simulink model "Model_pf_regulacije"  (R2024a)
settings: Solver=VariableStepAuto  StartTime=0.0  StopTime=Tsim  RelTol=1e-3
values from neighbouring files (symbols this model uses):
  Cv = [c1 c0]    [Model_pf_regulacije_eng.m]
  Fn = 50    [Model_pf_regulacije_eng.m]
  Lv = [l1 l0]    [Model_pf_regulacije_eng.m]
  n_LG2_CHM = 13    [Model_pf_regulacije_eng.m]
  n_LG2_LG3 = 2    [Model_pf_regulacije_eng.m]
  n_LG3_CHM = 6    [Model_pf_regulacije_eng.m]
  n_LG3_LG4 = 2    [Model_pf_regulacije_eng.m]
  n_LG4_CHM = 8    [Model_pf_regulacije_eng.m]
  P_LG31loc = 5e6    (= 5000000)    [Model_pf_regulacije_eng.m]
  PSStype = 1    [Model_pf_regulacije_eng.m]
  Rv = [r1 r0]    [Model_pf_regulacije_eng.m]
  t_ispad_LG31 = 100    [Model_pf_regulacije_eng.m]
  t_ispad_voda_LG2_LG3 = 1e6    (= 1000000)    [Model_pf_regulacije_eng.m]
  t_povecanje_potrosnje = 1e6    (= 1000000)    [Model_pf_regulacije_eng.m]
  Ts = 50e-6    (= 5e-05)    [Model_pf_regulacije_eng.m]
  Vg = 13.8e3    (= 13800)    [Model_pf_regulacije_eng.m]
  Vrms = 230e3    (= 230000)    [Model_pf_regulacije_eng.m]
undefined symbols (not defined in the file or in its folder): D1, Delta
libraries: spsThreePhaseParallelRLCLoadLib x6, spsDistributedParametersLineLib x5, spsThreePhaseTransformerTwoWindingsLib x4, spsSynchronousMachinepuStandardLib x4, spsRMSLib x4, spsExcitationSystemLib x4, spsHydraulicTurbineandGovernorLib x4, spsGenericPowerSystemStabilizerLib x4, spsMultiBandPowerSystemStabilizerLib x4, spsThreePhaseBreakerLib x3, spsThreePhaseSeriesRLCLoadLib x2, dspstat3 x2
(part 1 of 2)
settings Model: Creator=nesat  LastModifiedBy=nesat

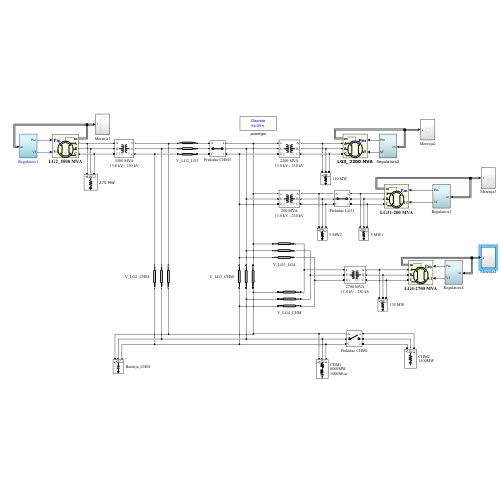
[thumbnail: Simulink's stored preview of the top-level diagram]
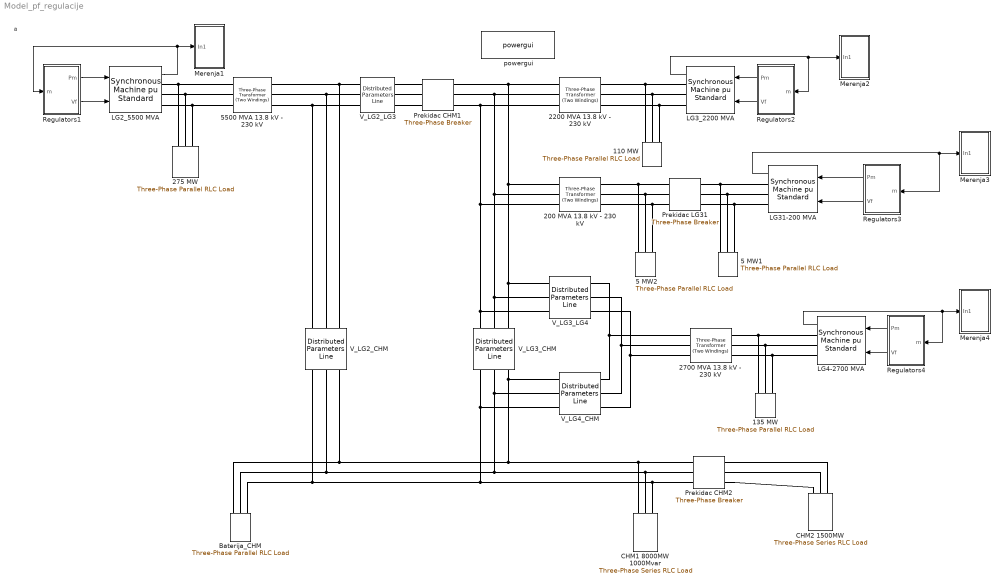
== system Model_pf_regulacije ==
  note: a
  110 MW : spsThreePhaseParallelRLCLoadLib/Three-Phase Parallel RLC Load  LConnTagsString=A|B|C  Configuration=Y (grounded)  NominalVoltage=(13800)*1  Vabc=[1e3 1e3 1e3]  Vabcp=[1e3 1e3 1e3]  NominalFrequency=Fn  UnbalancedPower=off  ActivePower=110000000  InductivePower=0  CapacitivePower=0  Pabc=[10e3 9e3 11e3]  QLabc=[100 90 110]  QCabc=[100 90 110]  Pabcp=[10e3 9e3 11e3]  QLabcp=[100 90 110]  QCabcp=[100 90 110]  Measurements=None  LoadType=constant PQ
  135 MW : spsThreePhaseParallelRLCLoadLib/Three-Phase Parallel RLC Load  LConnTagsString=A|B|C  Configuration=Y (grounded)  NominalVoltage=(13800)*1  Vabc=[1e3 1e3 1e3]  Vabcp=[1e3 1e3 1e3]  NominalFrequency=Fn  UnbalancedPower=off  ActivePower=135000000  InductivePower=0  CapacitivePower=0  Pabc=[10e3 9e3 11e3]  QLabc=[100 90 110]  QCabc=[100 90 110]  Pabcp=[10e3 9e3 11e3]  QLabcp=[100 90 110]  QCabcp=[100 90 110]  Measurements=None  LoadType=constant PQ
  200 MVA 13.8 kV - 230 kV : spsThreePhaseTransformerTwoWindingsLib/Three-Phase Transformer (Two Windings)  Winding1Connection=Delta (D1)  Winding2Connection=Yg  CoreType=Three single-phase transformers  SetSaturation=off  Hysteresis=off  DataFile='basic_model'  SetInitialFlux=off  Measurements=None  UNITS=pu  NominalPower=[ 200e6 Fn ]  Winding1="[ Vg 0.002  0.0]"  Winding2=[ Vrms 0.002 0.12]  Rm=500  Lm=500  L0=0.5  Saturation="[ 0,0  ;  0.005,1.2  ;  1.0,1.4 ]"  InitialFluxes=[ 0.8 , -0.8 , 0.7 ]  BreakLoop=off  DiscreteSolver=Trapezoidal iterative  DataType=off  TransfoNumber=0
  2200 MVA 13.8 kV - 230 kV : spsThreePhaseTransformerTwoWindingsLib/Three-Phase Transformer (Two Windings)  Winding1Connection=Delta (D1)  Winding2Connection=Yg  CoreType=Three single-phase transformers  SetSaturation=off  Hysteresis=off  DataFile='basic_model'  SetInitialFlux=off  Measurements=None  UNITS=pu  NominalPower=[ 2200e6 Fn ]  Winding1="[ Vg 0.002  0.0]"  Winding2=[ Vrms 0.002 0.12]  Rm=500  Lm=500  L0=0.5  Saturation="[ 0,0  ;  0.005,1.2  ;  1.0,1.4 ]"  InitialFluxes=[ 0.8 , -0.8 , 0.7 ]  BreakLoop=off  DiscreteSolver=Trapezoidal iterative  DataType=off  TransfoNumber=0
  2700 MVA 13.8 kV - 230 kV : spsThreePhaseTransformerTwoWindingsLib/Three-Phase Transformer (Two Windings)  Winding1Connection=Delta (D1)  Winding2Connection=Yg  CoreType=Three single-phase transformers  SetSaturation=off  Hysteresis=off  DataFile='basic_model'  SetInitialFlux=off  Measurements=None  UNITS=pu  NominalPower=[ 2700e6 Fn ]  Winding1="[ Vg 0.002  0.0]"  Winding2=[ Vrms 0.002 0.12]  Rm=500  Lm=500  L0=0.5  Saturation="[ 0,0  ;  0.005,1.2  ;  1.0,1.4 ]"  InitialFluxes=[ 0.8 , -0.8 , 0.7 ]  BreakLoop=off  DiscreteSolver=Trapezoidal iterative  DataType=off  TransfoNumber=0
  275 MW : spsThreePhaseParallelRLCLoadLib/Three-Phase Parallel RLC Load  LConnTagsString=A|B|C  Configuration=Y (grounded)  NominalVoltage=(13800)*1  Vabc=[1e3 1e3 1e3]  Vabcp=[1e3 1e3 1e3]  NominalFrequency=Fn  UnbalancedPower=off  ActivePower=275000000  InductivePower=0  CapacitivePower=0  Pabc=[10e3 9e3 11e3]  QLabc=[100 90 110]  QCabc=[100 90 110]  Pabcp=[10e3 9e3 11e3]  QLabcp=[100 90 110]  QCabcp=[100 90 110]  Measurements=None  LoadType=constant PQ
  5 MW1 : spsThreePhaseParallelRLCLoadLib/Three-Phase Parallel RLC Load  LConnTagsString=A|B|C  Configuration=Y (grounded)  NominalVoltage=(13800)*1  Vabc=[1e3 1e3 1e3]  Vabcp=[1e3 1e3 1e3]  NominalFrequency=Fn  UnbalancedPower=off  ActivePower=110000000  InductivePower=0  CapacitivePower=0  Pabc=[10e3 9e3 11e3]  QLabc=[100 90 110]  QCabc=[100 90 110]  Pabcp=[10e3 9e3 11e3]  QLabcp=[100 90 110]  QCabcp=[100 90 110]  Measurements=None  LoadType=constant PQ
  5 MW2 : spsThreePhaseParallelRLCLoadLib/Three-Phase Parallel RLC Load  LConnTagsString=A|B|C  Configuration=Y (grounded)  NominalVoltage=(13749.3)*1  Vabc=[1e3 1e3 1e3]  Vabcp=[1e3 1e3 1e3]  NominalFrequency=Fn  UnbalancedPower=off  ActivePower=110000000  InductivePower=0  CapacitivePower=0  Pabc=[10e3 9e3 11e3]  QLabc=[100 90 110]  QCabc=[100 90 110]  Pabcp=[10e3 9e3 11e3]  QLabcp=[100 90 110]  QCabcp=[100 90 110]  Measurements=None  LoadType=constant PQ
  5500 MVA 13.8 kV - 230 kV : spsThreePhaseTransformerTwoWindingsLib/Three-Phase Transformer (Two Windings)  Winding1Connection=Delta (D1)  Winding2Connection=Yg  CoreType=Three single-phase transformers  SetSaturation=off  Hysteresis=off  DataFile='basic_model'  SetInitialFlux=off  Measurements=None  UNITS=pu  NominalPower=[ 5500e6 Fn ]  Winding1="[ Vg 0.002  0.0]"  Winding2=[ Vrms 0.002 0.12]  Rm=500  Lm=500  L0=0.5  Saturation="[ 0,0  ;  0.005,1.2  ;  1.0,1.4 ]"  InitialFluxes=[ 0.8 , -0.8 , 0.7 ]  BreakLoop=off  DiscreteSolver=Trapezoidal iterative  DataType=off  TransfoNumber=0
  Baterija_CHM : spsThreePhaseParallelRLCLoadLib/Three-Phase Parallel RLC Load  LConnTagsString=A|B|C  Configuration=Y (grounded)  NominalVoltage=Vrms  Vabc=[1e3 1e3 1e3]  Vabcp=[1e3 1e3 1e3]  NominalFrequency=Fn  UnbalancedPower=off  ActivePower=0  InductivePower=0  CapacitivePower=2200000000  Pabc=[10e3 9e3 11e3]  QLabc=[100 90 110]  QCabc=[100 90 110]  Pabcp=[10e3 9e3 11e3]  QLabcp=[100 90 110]  QCabcp=[100 90 110]  Measurements=None  LoadType=constant Z
  CHM1 8000MW 1000Mvar : spsThreePhaseSeriesRLCLoadLib/Three-Phase Series RLC Load  LConnTagsString=A|B|C  Configuration=Y (grounded)  NominalVoltage=Vrms  Vabc=[1e3 1e3 1e3]  Vabcp=[1e3 1e3 1e3]  NominalFrequency=Fn  UnbalancedPower=off  ActivePower=8000000000  InductivePower=1000000000  CapacitivePower=0  Pabc=[10e3 9e3 11e3]  QLabc=[100 90 110]  QCabc=[100 90 110]  Pabcp=[10e3 9e3 11e3]  QLabcp=[100 90 110]  QCabcp=[100 90 110]  Measurements=None  LoadType=constant Z
  CHM2 1500MW : spsThreePhaseSeriesRLCLoadLib/Three-Phase Series RLC Load  LConnTagsString=A|B|C  Configuration=Y (grounded)  NominalVoltage=Vrms  Vabc=[1e3 1e3 1e3]  Vabcp=[1e3 1e3 1e3]  NominalFrequency=Fn  UnbalancedPower=off  ActivePower=1500000000  InductivePower=0  CapacitivePower=0  Pabc=[10e3 9e3 11e3]  QLabc=[100 90 110]  QCabc=[100 90 110]  Pabcp=[10e3 9e3 11e3]  QLabcp=[100 90 110]  QCabcp=[100 90 110]  Measurements=None  LoadType=constant Z
  LG2_5500 MVA : spsSynchronousMachinepuStandardLib/Synchronous Machine pu Standard  PresetModel=No  MechanicalLoad=Mechanical power Pm  ShowDetailedParameters=on  RotorType=Salient-pole  Units=per unit standard parameters  MeasurementBus=off  NominalParameters="[5500E6  Vg   Fn ]"  Reactances1=[ 31 32 33 34 35 36 37 ]  Reactances2=[ 1.305, 0.296, 0.252, 0.474, 0.243, 0.18 ]  dAxisTimeConstants=Short-circuit  qAxisTimeConstants=Open-circuit  TimeConstants1=[]  TimeConstants2=[]  TimeConstants3=[]  TimeConstants4=[]  TimeConstants5=[ 1.01, 0.053, 0.1 ]  TimeConstants6=[]  TimeConstants7=[]  TimeConstants8=[]  StatorResistance=2.8544e-3  Mechanical="[ 4.1  0  32]"  PolePairs=32  InitialConditions=[0 -70.1006 0.783509 0.783509 0.783509 -3.33907 -123.339 116.661 1.34578]  SetSaturation=off  Saturation=[0.6404,0.7127,0.8441,0.9214,0.9956,1.082,1.19,1.316,1.457;0.7,0.7698,0.8872,0.9466,0.9969,1.046,1.1,1.151,1.201]  LoadFlowParameters=[2 4000000000 0 0 0]  TsPowergui=0  TsBlock=-1  IterativeModel=Trapezoidal non iterative  IterativeDiscreteModel=Trapezoidal non iterative  BusType=swing  Pref=0  Qref=0  Qmin=-Inf  Qmax=Inf  PLF=0  QLF=0
  LG31-200 MVA : spsSynchronousMachinepuStandardLib/Synchronous Machine pu Standard  PresetModel=No  MechanicalLoad=Mechanical power Pm  ShowDetailedParameters=on  RotorType=Salient-pole  Units=per unit standard parameters  MeasurementBus=off  NominalParameters="[200E6  Vg   Fn ]"  Reactances1=[ 31 32 33 34 35 36 37 ]  Reactances2=[ 1.305, 0.296, 0.252, 0.474, 0.243, 0.18 ]  dAxisTimeConstants=Short-circuit  qAxisTimeConstants=Open-circuit  TimeConstants1=[]  TimeConstants2=[]  TimeConstants3=[]  TimeConstants4=[]  TimeConstants5=[ 1.01, 0.053, 0.1 ]  TimeConstants6=[]  TimeConstants7=[]  TimeConstants8=[]  StatorResistance=2.8544e-3  Mechanical="[ 3.2  0  32]"  PolePairs=32  InitialConditions=[0 -75.957 0.900232 0.900232 0.900232 -10.1077 -130.108 109.892 1.40453]  SetSaturation=off  Saturation=[0.6404,0.7127,0.8441,0.9214,0.9956,1.082,1.19,1.316,1.457;0.7,0.7698,0.8872,0.9466,0.9969,1.046,1.1,1.151,1.201]  LoadFlowParameters=[1 180000000 0 0 0]  TsPowergui=0  TsBlock=-1  IterativeModel=Trapezoidal non iterative  IterativeDiscreteModel=Trapezoidal non iterative  BusType=PV  Pref=180000000  Qref=0  Qmin=-Inf  Qmax=Inf  PLF=0  QLF=0
  LG3_2200 MVA : spsSynchronousMachinepuStandardLib/Synchronous Machine pu Standard  PresetModel=No  MechanicalLoad=Mechanical power Pm  ShowDetailedParameters=on  RotorType=Salient-pole  Units=per unit standard parameters  MeasurementBus=off  NominalParameters="[2200E6  Vg   Fn ]"  Reactances1=[ 31 32 33 34 35 36 37 ]  Reactances2=[ 1.305, 0.296, 0.252, 0.474, 0.243, 0.18 ]  dAxisTimeConstants=Short-circuit  qAxisTimeConstants=Open-circuit  TimeConstants1=[]  TimeConstants2=[]  TimeConstants3=[]  TimeConstants4=[]  TimeConstants5=[ 1.01, 0.053, 0.1 ]  TimeConstants6=[]  TimeConstants7=[]  TimeConstants8=[]  StatorResistance=2.8544e-3  Mechanical="[ 3.2  0  32]"  PolePairs=32  InitialConditions=[0 -71.4065 0.819807 0.819807 0.819807 -5.69934 -125.699 114.301 1.37781]  SetSaturation=off  Saturation=[0.6404,0.7127,0.8441,0.9214,0.9956,1.082,1.19,1.316,1.457;0.7,0.7698,0.8872,0.9466,0.9969,1.046,1.1,1.151,1.201]  LoadFlowParameters=[1 1800000000 0 0 0]  TsPowergui=0  TsBlock=-1  IterativeModel=Trapezoidal non iterative  IterativeDiscreteModel=Trapezoidal non iterative  BusType=PV  Pref=1800000000  Qref=0  Qmin=-Inf  Qmax=Inf  PLF=0  QLF=0
  LG4-2700 MVA : spsSynchronousMachinepuStandardLib/Synchronous Machine pu Standard  PresetModel=No  MechanicalLoad=Mechanical power Pm  ShowDetailedParameters=on  RotorType=Salient-pole  Units=per unit standard parameters  MeasurementBus=off  NominalParameters="[2700E6  Vg   Fn ]"  Reactances1=[ 31 32 33 34 35 36 37 ]  Reactances2=[ 1.305, 0.296, 0.252, 0.474, 0.243, 0.18 ]  dAxisTimeConstants=Short-circuit  qAxisTimeConstants=Open-circuit  TimeConstants1=[]  TimeConstants2=[]  TimeConstants3=[]  TimeConstants4=[]  TimeConstants5=[ 1.01, 0.053, 0.1 ]  TimeConstants6=[]  TimeConstants7=[]  TimeConstants8=[]  StatorResistance=2.8544e-3  Mechanical="[ 3.7  0  32]"  PolePairs=32  InitialConditions=[0 -69.3817 0.928059 0.928059 0.928059 -6.28858 -126.289 113.711 1.4708]  SetSaturation=off  Saturation=[0.6404,0.7127,0.8441,0.9214,0.9956,1.082,1.19,1.316,1.457;0.7,0.7698,0.8872,0.9466,0.9969,1.046,1.1,1.151,1.201]  LoadFlowParameters=[1 2500000000 0 0 0]  TsPowergui=0  TsBlock=-1  IterativeModel=Trapezoidal non iterative  IterativeDiscreteModel=Trapezoidal non iterative  BusType=PV  Pref=2500000000  Qref=0  Qmin=-Inf  Qmax=Inf  PLF=0  QLF=0
  Merenja1 : Subsystem
  Merenja2 : Subsystem
  Merenja3 : Subsystem
  Merenja4 : Subsystem
  Prekidac CHM1 : spsThreePhaseBreakerLib/Three-Phase Breaker  InitialState=closed  SwitchA=on  SwitchB=on  SwitchC=on  SwitchTimes=[t_ispad_voda_LG2_LG3]  External=off  BreakerResistance=0.01  SnubberResistance=inf  SnubberCapacitance=inf  Measurements=None
  Prekidac CHM2 : spsThreePhaseBreakerLib/Three-Phase Breaker  InitialState=open  SwitchA=on  SwitchB=on  SwitchC=on  SwitchTimes=[t_povecanje_potrosnje]  External=off  BreakerResistance=0.01  SnubberResistance=inf  SnubberCapacitance=inf  Measurements=None
  Prekidac LG31 : spsThreePhaseBreakerLib/Three-Phase Breaker  InitialState=closed  SwitchA=on  SwitchB=on  SwitchC=on  SwitchTimes=[t_ispad_LG31]  External=off  BreakerResistance=0.01  SnubberResistance=inf  SnubberCapacitance=inf  Measurements=None
  Regulators1 : Subsystem
  Regulators2 : Subsystem
  Regulators3 : Subsystem
  Regulators4 : Subsystem
  V_LG2_CHM : spsDistributedParametersLineLib/Distributed Parameters Line  Phases=3  Length=d_LG2_CHM  Frequency=Fn  Resistance=Rv/n_LG2_CHM  Inductance=Lv/n_LG2_CHM  Capacitance=Cv*n_LG2_CHM  x1=[-0.0004 -4.92231625974316e-10 0 0;-0.00035 -4.9297484247355e-10 0 0;-0.0003 -4.93596424806945e-10 174298.798867466 -148541.05620319;-0.00025 -4.9409621960836e-10 176610.478606358 -145784.962686328;-0.0002 -4.94474103560907e-10 178878.582352334 -142992.898911351;-0.00015 -4.94729983427376e-10 181102.550484731 -140165.553778216;-0.0001 -4.94863796073237e-10 183281.834272692 -137303.624892029;-5e-05 -4.94875508482223e-10 185415.896010552 -134407.818390917]  x2=[-0.0004 2.36773299637199e-10 0 0;-0.00035 2.32836541357427e-10 0 0;-0.0003 2.28842334145082e-10 144026.029759485 -176441.794650633;-0.00025 2.24791663511028e-10 146779.690253438 -174157.764140718;-0.0002 2.20685528897633e-10 149497.135055132 -171830.76280848;-0.00015 2.16524943432171e-10 152177.693675726 -169461.364806678;-0.0001 2.12310933676849e-10 154820.704727488 -167050.154748815;-5e-05 2.08044539375519e-10 157425.516086991 -164597.727564892]  x3=[-0.0004 3.21876795891022e-11 0 0;-0.00035 3.32508643823564e-11 0 0;-0.0003 3.43058450223675e-11 -6703.30163476618 5237.16864274642;-0.00025 3.53523612084488e-11 -6784.73607008563 5131.23180111232;-0.0002 3.63901547283906e-11 -6864.49647330198 5024.02890481155;-0.00015 3.74189695221708e-11 -6942.5631647292 4915.58640455469;-0.0001 3.84385517451334e-11 -7018.91688257933 4805.931056906;-5e-05 3.94486498306213e-11 -7093.53878771499 4695.08991768171]  x4=[-0.0004 -4.06922002783782e-11 0 0;-0.00035 -4.20487159660441e-11 0 0;-0.0003 -4.33948567622339e-11 17021.6965149512 -16716.63043995;-0.00025 -4.47302905268488e-11 17282.1696226858 -16447.2030111636;-0.0002 -4.60546877615899e-11 17538.3786136646 -16173.7174811389;-0.00015 -4.73677216912569e-11 17790.2602721529 -15896.2413283383;-0.0001 -4.8669068344375e-11 18037.7524501204 -15614.8430158504;-5e-05 -4.995840663313e-11 18280.7940825755 -15329.5919744984]  x5=0.000365161017096251  V1=ones(3,3)  V2=ones(3,3)  I1=ones(3,3)  I2=ones(3,3)  nHarmo=1  Measurements=None  Decoupling=on  VsMag0=[186984.075518439 186983.986127739 186984.058818565]  VrMag0=[185966.39343063 185966.327411481 185966.338035223]  VsAngle0=[24.9616648723654 -95.0383252221643 144.961693546538]  VrAngle0=[14.6240938483193 -105.375914115677 134.624107481573]  IsMag0=[6982.19028183256 6982.21077254924 6982.2073947194]  IrMag0=[19582.2755022873 19582.289528592 19582.2917657676]  IsAngle0=[-152.599793624276 87.400271448419 -32.5999067067536]  IrAngle0=[20.9180760110638 -99.0818927363708 140.918056096077]
      settings: AttributesFormatString=\n
  V_LG2_LG3 : spsDistributedParametersLineLib/Distributed Parameters Line  Phases=3  Length=d_LG2_LG3  Frequency=Fn  Resistance=Rv/n_LG2_LG3  Inductance=Lv/n_LG2_LG3  Capacitance=Cv*n_LG2_LG3  x1=[-0.0002 -4.94474103560907e-10 0 0;-0.00015 -4.94729983427376e-10 181102.550484731 -140165.553778216;-0.0001 -4.94863796073237e-10 183281.834272692 -137303.624892029;-5e-05 -4.94875508482223e-10 185415.896010552 -134407.818390917]  x2=[-0.0002 -7.7953967209642e-10 0 0;-0.00015 -7.86855540206448e-10 175151.457634006 -147384.64347033;-0.0001 -7.93977263485902e-10 177444.868089399 -144615.299555331;-5e-05 -8.00903084756128e-10 179694.496678755 -141810.273979092]  x3=[-0.0002 1.33778643921854e-11 0 0;-0.00015 1.31674782162147e-11 -28.2189110152237 -142.274491350519;-0.0001 1.29538431620234e-11 -25.9806898373746 -142.700175699615;-5e-05 1.27370119408644e-11 -23.7360583130655 -143.090650915626]  x4=[-0.0002 -1.7897483501798e-11 0 0;-0.00015 -1.77244134939981e-11 1861.28121044207 -1403.22806397395;-0.0001 -1.75469702523846e-11 1883.09255919525 -1373.81920400992;-5e-05 -1.73651975584223e-11 1904.43928303676 -1344.0713747142]  x5=0.000182580508548125  V1=ones(3,3)  V2=ones(3,3)  I1=ones(3,3)  I2=ones(3,3)  nHarmo=1  Measurements=None  Decoupling=on  VsMag0=[186984.075518439 186983.986127739 186984.058818565]  VrMag0=[186905.178173425 186905.084989887 186905.161229939]  VsAngle0=[24.9616648723654 -95.0383252221643 144.961693546538]  VrAngle0=[22.6203950553895 -97.3795944499093 142.620425041114]  IsMag0=[118.740998777895 118.740595365614 118.741154186562]  IrMag0=[1908.23825342973 1908.23711991417 1908.23756444361]  IsAngle0=[-38.5186191165268 -158.518420141088 81.4816489491208]  IrAngle0=[25.6871839847176 -94.3128202530022 145.687211340485]
      settings: AttributesFormatString=\n
  V_LG3_CHM : spsDistributedParametersLineLib/Distributed Parameters Line  Phases=3  Length=d_LG3_CHM  Frequency=Fn  Resistance=Rv/n_LG3_CHM  Inductance=Lv/n_LG3_CHM  Capacitance=Cv*n_LG3_CHM  x1=[-0.0003 3.60679163287581e-10 0 0;-0.00025 3.46849489679935e-10 170426.301829629 -152806.935817911;-0.0002 3.32934236150731e-10 172805.464821387 -150111.142456335;-0.00015 3.18936836080559e-10 175141.990650445 -147378.311416519;-0.0001 3.04860743118438e-10 177435.302814015 -144609.116983631;-5e-05 2.90709430329682e-10 179684.835471637 -141804.242414959]  x2=[-0.0003 5.63637905808929e-11 0 0;-0.00025 5.18487152588664e-11 146779.690253438 -174157.764140718;-0.0002 4.73208470421787e-11 149497.135055132 -171830.76280848;-0.00015 4.27813031145603e-11 152177.693675726 -169461.364806678;-0.0001 3.82312035405489e-11 154820.704727488 -167050.154748815;-5e-05 3.36716709891296e-11 157425.516086992 -164597.727564892]  x3=[-0.0003 -5.17988986960856e-11 0 0;-0.00025 -5.21005495720223e-11 -3261.95177657882 2594.96524324426;-0.0002 -5.23893454169493e-11 -3302.30898560715 2543.40867748096;-0.00015 -5.26652149748133e-11 -3341.85139930679 2491.22456368434;-0.0001 -5.29280901789288e-11 -3380.56926117886 2438.42577750362;-5e-05 -5.31779061687727e-11 -3418.45301817026 2385.02534624926]  x4=[-0.0003 5.38997922352836e-11 0 0;-0.00025 5.41154066451993e-11 8069.93383069662 -7880.48555179821;-0.0002 5.43176688882715e-11 8192.71927209322 -7752.75638122329;-0.00015 5.45065290593182e-11 8313.48328259971 -7623.11433401827;-0.0001 5.46819405599183e-11 8432.19606550355 -7491.59139741845;-5e-05 5.48438601099086e-11 8548.82833020188 -7358.2200227404]  x5=0.000273870762822188  V1=ones(3,3)  V2=ones(3,3)  I1=ones(3,3)  I2=ones(3,3)  nHarmo=1  Measurements=None  Decoupling=on  VsMag0=[186895.934962322 186895.841784948 186895.91802478]  VrMag0=[185966.39343063 185966.327411481 185966.338035223]  VsAngle0=[22.6200820806876 -97.3799074230796 142.620112066765]  VrAngle0=[14.6240938483193 -105.375914115677 134.624107481573]  IsMag0=[3416.77743069497 3416.79081502547 3416.789329226]  IrMag0=[9245.99519366939 9246.00534372241 9246.00684286608]  IsAngle0=[-154.003037127926 85.997063683 -34.0031810934756]  IrAngle0=[20.1805111179014 -99.819441840853 140.180480167284]
      settings: AttributesFormatString=\n
  V_LG3_LG4 : spsDistributedParametersLineLib/Distributed Parameters Line  Phases=3  Length=d_LG3_LG4  Frequency=Fn  Resistance=Rv/n_LG3_LG4  Inductance=Lv/n_LG3_LG4  Capacitance=Cv*n_LG3_LG4  x1=[-0.0002 3.32934236150731e-10 0 0;-0.00015 3.18936836080559e-10 175141.990650445 -147378.311416519;-0.0001 3.04860743118438e-10 177435.302814015 -144609.116983631;-5e-05 2.90709430329682e-10 179684.835471637 -141804.242414959]  x2=[-0.0002 1.21043284557454e-10 0 0;-0.00015 1.09009725018709e-10 172295.654093928 -150519.718237425;-0.0001 9.69492689614629e-11 174638.661520085 -147794.848187023;-5e-05 8.48648921227839e-11 176938.579469686 -145033.511969331]  x3=[-0.0002 -6.1608129553596e-12 0 0;-0.00015 -6.39604605721854e-12 478.611469515026 -493.959673085078;-0.0001 -6.62970103041895e-12 486.311664006773 -486.380949799821;-5e-05 -6.86172022409245e-12 493.891868372263 -478.682219293075]  x4=[-0.0002 5.42735736797522e-12 0 0;-0.00015 5.47118398448572e-12 1307.12976761467 -1104.73436688628;-0.0001 5.51366066821513e-12 1324.32048212396 -1084.06665754206;-5e-05 5.55477693867734e-12 1341.18444037052 -1063.13147097132]  x5=0.000182580508548125  V1=ones(3,3)  V2=ones(3,3)  I1=ones(3,3)  I2=ones(3,3)  nHarmo=1  Measurements=None  Decoupling=on  VsMag0=[186895.934962322 186895.841784948 186895.91802478]  VrMag0=[186801.151920291 186801.129926176 186801.036069883]  VsAngle0=[22.6200820806876 -97.3799074230796 142.620112066765]  VrAngle0=[21.5591107129978 -98.4409264229707 141.559097987269]  IsMag0=[563.084208908888 563.067141562085 563.065053621451]  IrMag0=[1401.04156139632 1401.05913786973 1401.05906764344]  IsAngle0=[16.7953210422352 -103.205926979985 136.796201085146]  IrAngle0=[22.4971326327252 -97.502455694665 142.496715985794]
      settings: AttributesFormatString=\n
  V_LG4_CHM : spsDistributedParametersLineLib/Distributed Parameters Line  Phases=3  Length=d_LG4_CHM  Frequency=Fn  Resistance=Rv/n_LG4_CHM  Inductance=Lv/n_LG4_CHM  Capacitance=Cv*n_LG4_CHM  x1=[-0.00025 1.33332411004425e-10 0 0;-0.0002 1.21271715136788e-10 169910.135293239 -153207.449799628;-0.00015 1.09181097288068e-10 172295.654093928 -150519.718237425;-0.0001 9.70635406373038e-11 174638.661520085 -147794.848187023;-5e-05 8.49220350102806e-11 176938.579469686 -145033.511969331]  x2=[-0.00025 5.18487152588664e-11 0 0;-0.0002 4.73208470421787e-11 149497.135055132 -171830.76280848;-0.00015 4.27813031145603e-11 152177.693675726 -169461.364806678;-0.0001 3.82312035405489e-11 154820.704727488 -167050.154748815;-5e-05 3.36716709891296e-11 157425.516086992 -164597.727564892]  x3=[-0.00025 -6.35851188186883e-11 0 0;-0.0002 -6.37198904871654e-11 -4698.16701989244 3704.41558440375;-0.00015 -6.38389402261261e-11 -4755.77476748485 3630.1627630419;-0.0001 -6.39422386618285e-11 -4812.20909881558 3555.01425333756;-5e-05 -6.40297603069293e-11 -4867.4560895578 3478.98859706102]  x4=[-0.00025 6.15787065574911e-11 0 0;-0.0002 6.13911826988325e-11 11198.9922638145 -10684.0251642951;-0.00015 6.1188511484459e-11 11365.4290381183 -10506.8007786139;-0.0001 6.097074292046e-11 11529.0615628715 -10326.9839970573;-5e-05 6.07379307379701e-11 11689.8494641972 -10144.6191867253]  x5=0.000228225635685157  V1=ones(3,3)  V2=ones(3,3)  I1=ones(3,3)  I2=ones(3,3)  nHarmo=1  Measurements=None  Decoupling=on  VsMag0=[186801.151920291 186801.129926176 186801.036069883]  VrMag0=[185966.39343063 185966.327411481 185966.338035223]  VsAngle0=[21.5591107129978 -98.4409264229707 141.559097987269]  VrAngle0=[14.6240938483193 -105.375914115677 134.624107481573]  IsMag0=[4901.16218584666 4901.12357747519 4901.1273090217]  IrMag0=[12679.2991118077 12679.2604661038 12679.2586149061]  IsAngle0=[-154.655313098145 85.3444766887383 -34.655027328508]  IrAngle0=[19.9480135573877 -100.05209692731 139.948109553019]
      settings: AttributesFormatString=\n
  powergui : spspowerguiLib/powergui  Priority=1  SimulationMode=Discrete  SampleTime=Ts  frequency=Fn  Iterations=50  frequencyindice=Fn  Pbase=Sbase  ErrMax=0.0001  UnitsV=kV  UnitsW=MW  buscounter=0  FunctionMessages=off  echomessages=off  EnableUseOfTLC=off  CurrentSourceSwitches=off  DisableSnubberDevices=off  DisableRonSwitches=off  DisableVfSwitches=off  DisplayEquations=off  AutomaticDiscreteSolvers=off  SolverType=Tustin/Backward Euler (TBE)  Interpol=off  ExternalGateDelay=off  methode=off  Ts=100  x0status=blocks  SPID=on  SwTol=0  HookPort=off  NonlinearTolerance=1e-4  nMaxIteration=100  ContinueOnMaxIteration=off  RestoreLinks=warning  ResistiveCurrentMeasurement=off  Frange=[0:2:500]  Ylog=off  Xlog=on  ShowGrid=off  save=off  variable=ZData  structure=0  ZoomFFT=off  StartTime=0.0  cycles=1  DisplayStyle=1  fundamental=Fn  FreqAxis=off  MaxFrequency=1000  frequencyindicesteady=1  RmsSteady=1  display=off
  wires:
  LG2_5500 MVA/1 -> Merenja1/1(In1), Regulators1/1(m)
  Regulators1/1(Pm) -> LG2_5500 MVA/1
  LG4-2700 MVA/1 -> Merenja4/1(In1), Regulators4/1(m)
  Regulators2/2(Vf) -> LG3_2200 MVA/2
  Regulators2/1(Pm) -> LG3_2200 MVA/1
  Regulators1/2(Vf) -> LG2_5500 MVA/2
  Regulators3/1(Pm) -> LG31-200 MVA/1
  Regulators4/2(Vf) -> LG4-2700 MVA/2
  Regulators4/1(Pm) -> LG4-2700 MVA/1
  Regulators3/2(Vf) -> LG31-200 MVA/2
  LG3_2200 MVA/1 -> Regulators2/1(m), Merenja2/1(In1)
  LG31-200 MVA/1 -> Merenja3/1(In1), Regulators3/1(m)
  connections:
  V_LG3_LG4/RConn1 -- 2700 MVA 13.8 kV - 230 kV/RConn1 -- V_LG4_CHM/LConn1
  LG3_2200 MVA/RConn2 -- 2200 MVA 13.8 kV - 230 kV/LConn2 -- 110 MW/LConn2
  V_LG4_CHM/RConn2 -- Prekidac CHM2/LConn2 -- CHM1 8000MW 1000Mvar/LConn2 -- V_LG2_CHM/RConn2 -- Baterija_CHM/LConn2 -- V_LG3_CHM/RConn2
  V_LG2_LG3/LConn3 -- 5500 MVA 13.8 kV - 230 kV/RConn3 -- V_LG2_CHM/LConn3
  V_LG3_LG4/LConn2 -- 200 MVA 13.8 kV - 230 kV/RConn2 -- Prekidac CHM1/RConn2 -- 2200 MVA 13.8 kV - 230 kV/RConn2 -- V_LG3_CHM/LConn2
  2700 MVA 13.8 kV - 230 kV/LConn1 -- LG4-2700 MVA/RConn1 -- 135 MW/LConn1
  2700 MVA 13.8 kV - 230 kV/LConn2 -- 135 MW/LConn2 -- LG4-2700 MVA/RConn2
  2700 MVA 13.8 kV - 230 kV/LConn3 -- LG4-2700 MVA/RConn3 -- 135 MW/LConn3
  LG3_2200 MVA/RConn3 -- 2200 MVA 13.8 kV - 230 kV/LConn3 -- 110 MW/LConn3
  V_LG3_LG4/RConn3 -- 2700 MVA 13.8 kV - 230 kV/RConn3 -- V_LG4_CHM/LConn3
  Prekidac CHM2/LConn3 -- CHM1 8000MW 1000Mvar/LConn3 -- V_LG2_CHM/RConn3 -- Baterija_CHM/LConn3 -- V_LG3_CHM/RConn3 -- V_LG4_CHM/RConn3
  V_LG4_CHM/RConn1 -- V_LG2_CHM/RConn1 -- Baterija_CHM/LConn1 -- CHM1 8000MW 1000Mvar/LConn1 -- Prekidac CHM2/LConn1 -- V_LG3_CHM/RConn1
  V_LG3_LG4/RConn2 -- 2700 MVA 13.8 kV - 230 kV/RConn2 -- V_LG4_CHM/LConn2
  V_LG2_LG3/LConn2 -- 5500 MVA 13.8 kV - 230 kV/RConn2 -- V_LG2_CHM/LConn2
  LG3_2200 MVA/RConn1 -- 2200 MVA 13.8 kV - 230 kV/LConn1 -- 110 MW/LConn1
  5500 MVA 13.8 kV - 230 kV/LConn3 -- LG2_5500 MVA/RConn3 -- 275 MW/LConn3
  V_LG3_LG4/LConn1 -- 2200 MVA 13.8 kV - 230 kV/RConn1 -- Prekidac CHM1/RConn1 -- 200 MVA 13.8 kV - 230 kV/RConn1 -- V_LG3_CHM/LConn1
  5500 MVA 13.8 kV - 230 kV/LConn1 -- LG2_5500 MVA/RConn1 -- 275 MW/LConn1
  5500 MVA 13.8 kV - 230 kV/LConn2 -- LG2_5500 MVA/RConn2 -- 275 MW/LConn2
  V_LG2_LG3/LConn1 -- 5500 MVA 13.8 kV - 230 kV/RConn1 -- V_LG2_CHM/LConn1
  V_LG3_CHM/LConn3 -- V_LG3_LG4/LConn3 -- Prekidac CHM1/RConn3 -- 2200 MVA 13.8 kV - 230 kV/RConn3 -- 200 MVA 13.8 kV - 230 kV/RConn3
  Prekidac CHM2/RConn1 -- CHM2 1500MW/LConn3
  Prekidac CHM2/RConn2 -- CHM2 1500MW/LConn2
  Prekidac CHM2/RConn3 -- CHM2 1500MW/LConn1
  Prekidac CHM1/LConn1 -- V_LG2_LG3/RConn1
  Prekidac CHM1/LConn2 -- V_LG2_LG3/RConn2
  Prekidac CHM1/LConn3 -- V_LG2_LG3/RConn3
  5 MW2/LConn1 -- 200 MVA 13.8 kV - 230 kV/LConn1 -- Prekidac LG31/LConn1
  Prekidac LG31/LConn2 -- 200 MVA 13.8 kV - 230 kV/LConn2 -- 5 MW2/LConn2
  5 MW2/LConn3 -- 200 MVA 13.8 kV - 230 kV/LConn3 -- Prekidac LG31/LConn3
  Prekidac LG31/RConn1 -- 5 MW1/LConn1 -- LG31-200 MVA/RConn1
  Prekidac LG31/RConn2 -- 5 MW1/LConn2 -- LG31-200 MVA/RConn2
  Prekidac LG31/RConn3 -- LG31-200 MVA/RConn3 -- 5 MW1/LConn3

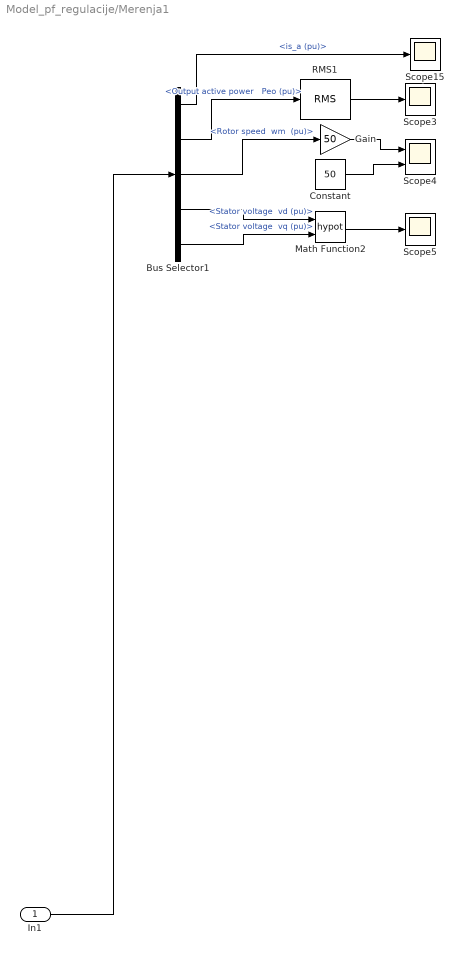
== system Model_pf_regulacije/Merenja1 ==
  In1 : Inport
  Bus Selector1 : BusSelector  OutputSignals="Stator current.is_a (pu),Output active power   Peo (pu),Mechanical.Rotor speed  wm  (pu),dq0 components.Stator voltage  vd (pu),dq0 components.Stator voltage  vq (pu)"
  Constant : Constant  Value=50
  Gain : Gain  Gain=50
  Math Function2 : Math  Operator=hypot  SignedPower=on
  RMS1 : spsRMSLib/RMS  TrueRMS=on  Freq=50  RMSInit=0.6  Ts=0
  Scope15 : Scope
  Scope3 : Scope
  Scope4 : Scope  NumInputPorts=2
  Scope5 : Scope
  wires:
  RMS1/1 -> Scope3/1
  Bus Selector1/2 -> RMS1/1  "<Output active power   Peo (pu)>"
  Bus Selector1/5 -> Math Function2/2  "<Stator voltage  vq (pu)>"
  Gain/1 -> Scope4/1
  Bus Selector1/3 -> Gain/1  "<Rotor speed  wm  (pu)>"
  Constant/1 -> Scope4/2
  In1/1 -> Bus Selector1/1
  Bus Selector1/1 -> Scope15/1  "<is_a (pu)>"
  Bus Selector1/4 -> Math Function2/1  "<Stator voltage  vd (pu)>"
  Math Function2/1 -> Scope5/1

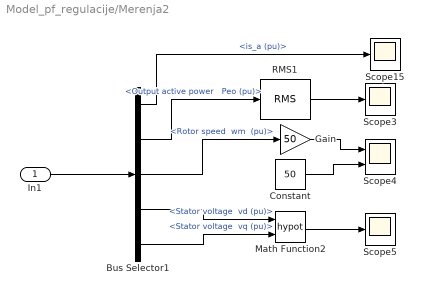
== system Model_pf_regulacije/Merenja2 ==
  In1 : Inport
  Bus Selector1 : BusSelector  OutputSignals="Stator current.is_a (pu),Output active power   Peo (pu),Mechanical.Rotor speed  wm  (pu),dq0 components.Stator voltage  vd (pu),dq0 components.Stator voltage  vq (pu)"
  Constant : Constant  Value=50
  Gain : Gain  Gain=50
  Math Function2 : Math  Operator=hypot  SignedPower=on
  RMS1 : spsRMSLib/RMS  TrueRMS=on  Freq=50  RMSInit=0.6  Ts=0
  Scope15 : Scope
  Scope3 : Scope
  Scope4 : Scope  NumInputPorts=2
  Scope5 : Scope
  wires:
  Math Function2/1 -> Scope5/1
  Gain/1 -> Scope4/1
  In1/1 -> Bus Selector1/1
  Bus Selector1/3 -> Gain/1  "<Rotor speed  wm  (pu)>"
  Bus Selector1/5 -> Math Function2/2  "<Stator voltage  vq (pu)>"
  Bus Selector1/1 -> Scope15/1  "<is_a (pu)>"
  Bus Selector1/4 -> Math Function2/1  "<Stator voltage  vd (pu)>"
  Constant/1 -> Scope4/2
  RMS1/1 -> Scope3/1
  Bus Selector1/2 -> RMS1/1  "<Output active power   Peo (pu)>"

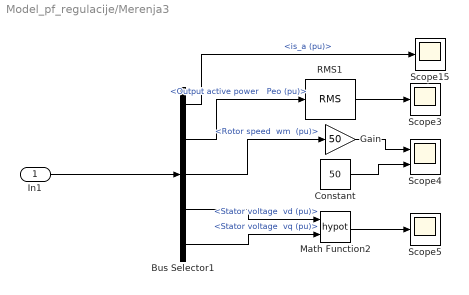
== system Model_pf_regulacije/Merenja3 ==
  In1 : Inport
  Bus Selector1 : BusSelector  OutputSignals="Stator current.is_a (pu),Output active power   Peo (pu),Mechanical.Rotor speed  wm  (pu),dq0 components.Stator voltage  vd (pu),dq0 components.Stator voltage  vq (pu)"
  Constant : Constant  Value=50
  Gain : Gain  Gain=50
  Math Function2 : Math  Operator=hypot  SignedPower=on
  RMS1 : spsRMSLib/RMS  TrueRMS=on  Freq=50  RMSInit=0.6  Ts=0
  Scope15 : Scope
  Scope3 : Scope
  Scope4 : Scope  NumInputPorts=2
  Scope5 : Scope
  wires:
  Math Function2/1 -> Scope5/1
  Gain/1 -> Scope4/1
  In1/1 -> Bus Selector1/1
  Bus Selector1/3 -> Gain/1  "<Rotor speed  wm  (pu)>"
  Bus Selector1/5 -> Math Function2/2  "<Stator voltage  vq (pu)>"
  Bus Selector1/1 -> Scope15/1  "<is_a (pu)>"
  Bus Selector1/4 -> Math Function2/1  "<Stator voltage  vd (pu)>"
  Constant/1 -> Scope4/2
  RMS1/1 -> Scope3/1
  Bus Selector1/2 -> RMS1/1  "<Output active power   Peo (pu)>"

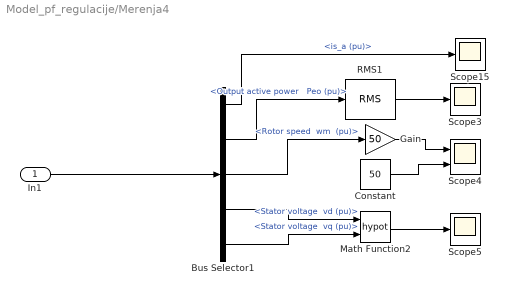
== system Model_pf_regulacije/Merenja4 ==
  In1 : Inport
  Bus Selector1 : BusSelector  OutputSignals="Stator current.is_a (pu),Output active power   Peo (pu),Mechanical.Rotor speed  wm  (pu),dq0 components.Stator voltage  vd (pu),dq0 components.Stator voltage  vq (pu)"
  Constant : Constant  Value=50
  Gain : Gain  Gain=50
  Math Function2 : Math  Operator=hypot  SignedPower=on
  RMS1 : spsRMSLib/RMS  TrueRMS=on  Freq=50  RMSInit=0.6  Ts=0
  Scope15 : Scope
  Scope3 : Scope
  Scope4 : Scope  NumInputPorts=2
  Scope5 : Scope
  wires:
  Math Function2/1 -> Scope5/1
  Gain/1 -> Scope4/1
  In1/1 -> Bus Selector1/1
  Bus Selector1/3 -> Gain/1  "<Rotor speed  wm  (pu)>"
  Bus Selector1/5 -> Math Function2/2  "<Stator voltage  vq (pu)>"
  Bus Selector1/1 -> Scope15/1  "<is_a (pu)>"
  Bus Selector1/4 -> Math Function2/1  "<Stator voltage  vd (pu)>"
  Constant/1 -> Scope4/2
  RMS1/1 -> Scope3/1
  Bus Selector1/2 -> RMS1/1  "<Output active power   Peo (pu)>"

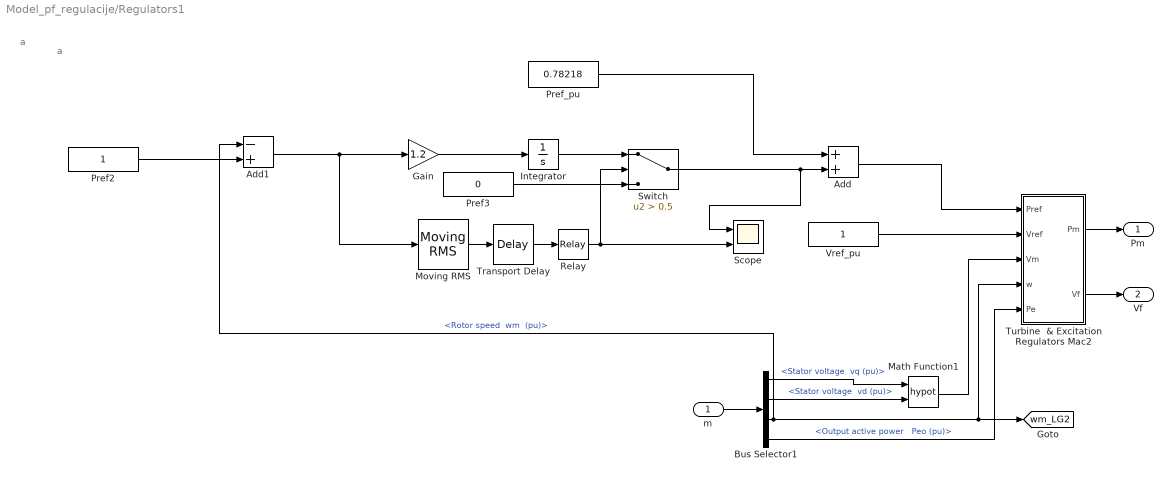
== system Model_pf_regulacije/Regulators1 ==
  note: a
  note: a
  m : Inport
  Add : Sum
  Add1 : Sum  Inputs=-+
  Bus Selector1 : BusSelector  OutputSignals="dq0 components.Stator voltage  vq (pu),dq0 components.Stator voltage  vd (pu),Mechanical.Rotor speed  wm  (pu),Output active power   Peo (pu)"
  Gain : Gain  Gain=1.2
  Integrator : Integrator  LimitOutput=on  UpperSaturationLimit=0.2  LowerSaturationLimit=-0.2
  Math Function1 : Math  Operator=hypot  SignedPower=on
  Moving RMS : dspstat3/Moving RMS  Method=Sliding window  ForgettingFactorPort=off  SpecifyWindowLength=on  WindowLength=4  OverlapLength=3  AllowArbitraryInputLength=off  ForgettingFactor=0.9  SimulateUsing=Interpreted execution
  Pref2 : Constant
  Pref3 : Constant  Value=0
  Pref_pu : Constant  Value=0.78218
  Relay : Relay  OnSwitchValue=0.0005  OffSwitchValue=0
  Scope : Scope  NumInputPorts=2
  Switch : Switch  Criteria=u2 > Threshold  Threshold=0.5  SaturateOnIntegerOverflow=off  InputSameDT=off
  Transport Delay : TransportDelay  DelayTime=65  BufferSize=1300480
  Turbine  & Excitation Regulators Mac2 : Subsystem
  Vref_pu : Constant
  Pm : Outport  VectorParamsAs1DForOutWhenUnconnected=off
  Vf : Outport  Port=2  VectorParamsAs1DForOutWhenUnconnected=off
  tag scope: wm_LG2=global
  wires:
  m/1 -> Bus Selector1/1
  Bus Selector1/4 -> Turbine  & Excitation Regulators Mac2/5(Pe)  "<Output active power   Peo (pu)>"
  Bus Selector1/3 -> Add1/1, [wm_LG2], Turbine  & Excitation Regulators Mac2/4(w)  "<Rotor speed  wm  (pu)>"
  Math Function1/1 -> Turbine  & Excitation Regulators Mac2/3(Vm)
  Bus Selector1/2 -> Math Function1/2  "<Stator voltage  vd (pu)>"
  Bus Selector1/1 -> Math Function1/1  "<Stator voltage  vq (pu)>"
  Turbine  & Excitation Regulators Mac2/2(Vf) -> Vf/1
  Turbine  & Excitation Regulators Mac2/1(Pm) -> Pm/1
  Vref_pu/1 -> Turbine  & Excitation Regulators Mac2/2(Vref)
  Gain/1 -> Integrator/1
  Pref2/1 -> Add1/2
  Pref3/1 -> Switch/3
  Integrator/1 -> Switch/1
  Switch/1 -> Scope/1, Add/2
  Add1/1 -> Moving RMS/1, Gain/1
  Relay/1 -> Scope/2, Switch/2
  Moving RMS/1 -> Transport Delay/1
  Transport Delay/1 -> Relay/1
  Pref_pu/1 -> Add/1
  Add/1 -> Turbine  & Excitation Regulators Mac2/1(Pref)

== system Model_pf_regulacije/Regulators2 ==
  note: a
  m : Inport
  Bus Selector1 : BusSelector  OutputSignals="dq0 components.Stator voltage  vq (pu),dq0 components.Stator voltage  vd (pu),Mechanical.Rotor speed  wm  (pu),Output active power   Peo (pu)"
  Math Function1 : Math  Operator=hypot  SignedPower=on
  Pref_pu : Constant  Value=0.81818
  Turbine  & Excitation Regulators Mac2 : Subsystem
  Vref_pu : Constant
  Pm : Outport  VectorParamsAs1DForOutWhenUnconnected=off
  Vf : Outport  Port=2  VectorParamsAs1DForOutWhenUnconnected=off
  tag scope: wm_LG3=global
  wires:
  Turbine  & Excitation Regulators Mac2/1(Pm) -> Pm/1
  Turbine  & Excitation Regulators Mac2/2(Vf) -> Vf/1
  Bus Selector1/1 -> Math Function1/1  "<Stator voltage  vq (pu)>"
  Bus Selector1/2 -> Math Function1/2  "<Stator voltage  vd (pu)>"
  Math Function1/1 -> Turbine  & Excitation Regulators Mac2/3(Vm)
  Bus Selector1/4 -> Turbine  & Excitation Regulators Mac2/5(Pe)  "<Output active power   Peo (pu)>"
  m/1 -> Bus Selector1/1
  Bus Selector1/3 -> [wm_LG3], Turbine  & Excitation Regulators Mac2/4(w)  "<Rotor speed  wm  (pu)>"
  Vref_pu/1 -> Turbine  & Excitation Regulators Mac2/2(Vref)
  Pref_pu/1 -> Turbine  & Excitation Regulators Mac2/1(Pref)

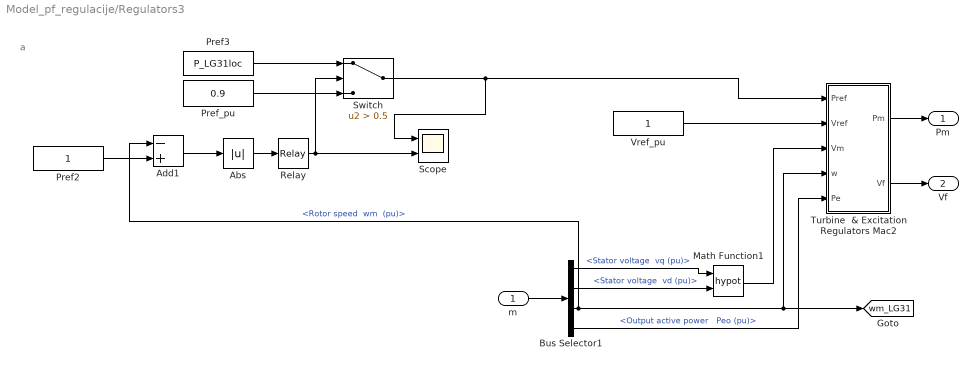
== system Model_pf_regulacije/Regulators3 ==
  note: a
  m : Inport
  Abs : Abs  SaturateOnIntegerOverflow=off
  Add1 : Sum  Inputs=-+
  Bus Selector1 : BusSelector  OutputSignals="dq0 components.Stator voltage  vq (pu),dq0 components.Stator voltage  vd (pu),Mechanical.Rotor speed  wm  (pu),Output active power   Peo (pu)"
  Math Function1 : Math  Operator=hypot  SignedPower=on
  Pref2 : Constant
  Pref3 : Constant  Value=P_LG31loc
  Pref_pu : Constant  Value=0.9
  Relay : Relay  OnSwitchValue=0.04  OffSwitchValue=-1  OnOutputValue=0.5
  Scope : Scope  NumInputPorts=2
  Switch : Switch  Criteria=u2 > Threshold  Threshold=0.5  SaturateOnIntegerOverflow=off  InputSameDT=off
  Turbine  & Excitation Regulators Mac2 : Subsystem
  Vref_pu : Constant
  Pm : Outport  VectorParamsAs1DForOutWhenUnconnected=off
  Vf : Outport  Port=2  VectorParamsAs1DForOutWhenUnconnected=off
  tag scope: wm_LG31=global
  wires:
  m/1 -> Bus Selector1/1
  Bus Selector1/4 -> Turbine  & Excitation Regulators Mac2/5(Pe)  "<Output active power   Peo (pu)>"
  Bus Selector1/3 -> Add1/1, [wm_LG31], Turbine  & Excitation Regulators Mac2/4(w)  "<Rotor speed  wm  (pu)>"
  Math Function1/1 -> Turbine  & Excitation Regulators Mac2/3(Vm)
  Bus Selector1/2 -> Math Function1/2  "<Stator voltage  vd (pu)>"
  Bus Selector1/1 -> Math Function1/1  "<Stator voltage  vq (pu)>"
  Turbine  & Excitation Regulators Mac2/2(Vf) -> Vf/1
  Turbine  & Excitation Regulators Mac2/1(Pm) -> Pm/1
  Vref_pu/1 -> Turbine  & Excitation Regulators Mac2/2(Vref)
  Pref_pu/1 -> Switch/3
  Abs/1 -> Relay/1
  Pref3/1 -> Switch/1
  Add1/1 -> Abs/1
  Pref2/1 -> Add1/2
  Relay/1 -> Scope/2, Switch/2
  Switch/1 -> Turbine  & Excitation Regulators Mac2/1(Pref), Scope/1

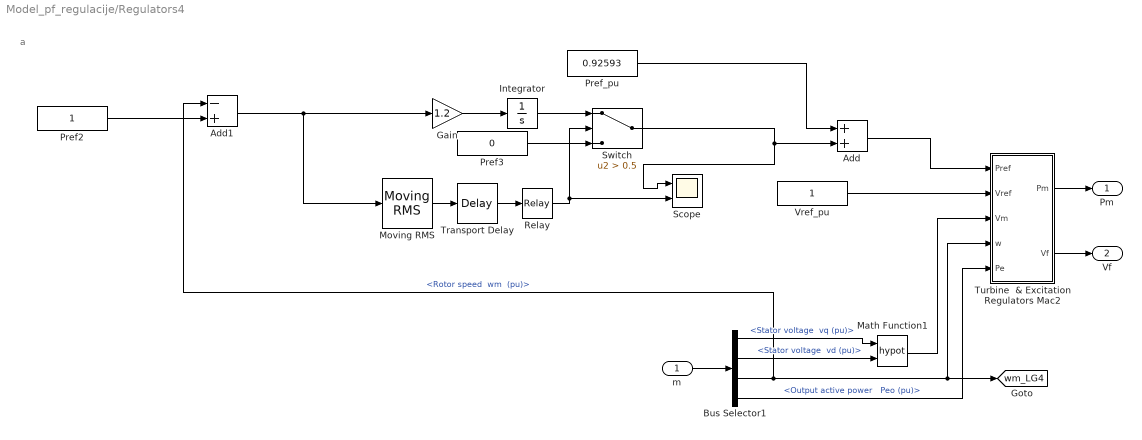
== system Model_pf_regulacije/Regulators4 ==
  note: a
  m : Inport
  Add : Sum
  Add1 : Sum  Inputs=-+
  Bus Selector1 : BusSelector  OutputSignals="dq0 components.Stator voltage  vq (pu),dq0 components.Stator voltage  vd (pu),Mechanical.Rotor speed  wm  (pu),Output active power   Peo (pu)"
  Gain : Gain  Gain=1.2
  Integrator : Integrator  LimitOutput=on  UpperSaturationLimit=0.1  LowerSaturationLimit=-0.1
  Math Function1 : Math  Operator=hypot  SignedPower=on
  Moving RMS : dspstat3/Moving RMS  Method=Sliding window  ForgettingFactorPort=off  SpecifyWindowLength=on  WindowLength=4  OverlapLength=3  AllowArbitraryInputLength=off  ForgettingFactor=0.9  SimulateUsing=Interpreted execution
  Pref2 : Constant
  Pref3 : Constant  Value=0
  Pref_pu : Constant  Value=0.92593
  Relay : Relay  OnSwitchValue=0.0005  OffSwitchValue=0
  Scope : Scope  NumInputPorts=2
  Switch : Switch  Criteria=u2 > Threshold  Threshold=0.5  SaturateOnIntegerOverflow=off  InputSameDT=off
  Transport Delay : TransportDelay  DelayTime=65  BufferSize=1300480
  Turbine  & Excitation Regulators Mac2 : Subsystem
  Vref_pu : Constant
  Pm : Outport  VectorParamsAs1DForOutWhenUnconnected=off
  Vf : Outport  Port=2  VectorParamsAs1DForOutWhenUnconnected=off
  tag scope: wm_LG4=global
  wires:
  Vref_pu/1 -> Turbine  & Excitation Regulators Mac2/2(Vref)
  Turbine  & Excitation Regulators Mac2/1(Pm) -> Pm/1
  Turbine  & Excitation Regulators Mac2/2(Vf) -> Vf/1
  Bus Selector1/1 -> Math Function1/1  "<Stator voltage  vq (pu)>"
  Bus Selector1/2 -> Math Function1/2  "<Stator voltage  vd (pu)>"
  Math Function1/1 -> Turbine  & Excitation Regulators Mac2/3(Vm)
  Bus Selector1/4 -> Turbine  & Excitation Regulators Mac2/5(Pe)  "<Output active power   Peo (pu)>"
  m/1 -> Bus Selector1/1
  Relay/1 -> Scope/2, Switch/2
  Add1/1 -> Moving RMS/1, Gain/1
  Switch/1 -> Add/2, Scope/1
  Transport Delay/1 -> Relay/1
  Pref3/1 -> Switch/3
  Gain/1 -> Integrator/1
  Moving RMS/1 -> Transport Delay/1
  Bus Selector1/3 -> Add1/1, Turbine  & Excitation Regulators Mac2/4(w), [wm_LG4]  "<Rotor speed  wm  (pu)>"
  Pref2/1 -> Add1/2
  Integrator/1 -> Switch/1
  Pref_pu/1 -> Add/1
  Add/1 -> Turbine  & Excitation Regulators Mac2/1(Pref)

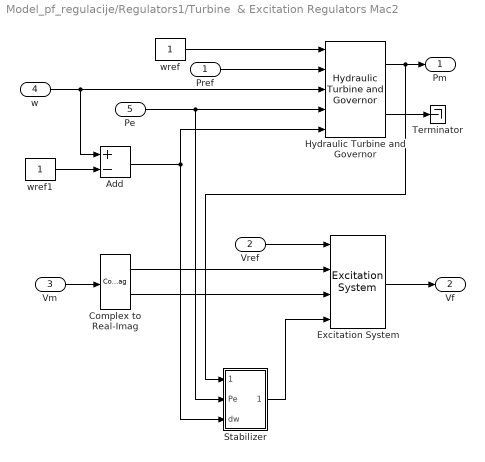
== system Model_pf_regulacije/Regulators1/Turbine  & Excitation Regulators Mac2 ==
  Pref : Inport
  Vref : Inport  Port=2
  Vm : Inport  Port=3
  w : Inport  Port=4
  Pe : Inport  Port=5
  Add : Sum  Inputs=+-
  Complex to Real-Imag : ComplexToRealImag
  Excitation System : spsExcitationSystemLib/Excitation System  tr=20e-3  reg=[ 300, 0.001 ]  exc=[ 1, 0 ]  tgr=[ 0, 0 ]  damp=[ 0.001, 0.1 ]  sat=[ 0, 0 ]  lim=[ -11.5, 11.5, 0 ]  v0=[1 1.3458]
  Hydraulic Turbine and Governor : spsHydraulicTurbineandGovernorLib/Hydraulic Turbine and Governor  sm="[ 10/3  0.07 ]"  gate="[  0.01  0.97518  -0.1  0.1 ]"  reg="[  0.05 1.163  0.105  0  0.01  ]"  hyd="[  0  2.67  ]"  dref=0  po=0.78393
  Stabilizer : Subsystem
  Terminator : Terminator
  wref : Constant
  wref1 : Constant
  Pm : Outport  VectorParamsAs1DForOutWhenUnconnected=off
  Vf : Outport  Port=2  VectorParamsAs1DForOutWhenUnconnected=off
  wires:
  Stabilizer/1(Stab) -> Excitation System/4
  Add/1 -> Stabilizer/3(dw), Hydraulic Turbine and Governor/5
  wref1/1 -> Add/2
  Complex to Real-Imag/1 -> Excitation System/2
  Complex to Real-Imag/2 -> Excitation System/3
  Vm/1 -> Complex to Real-Imag/1
  w/1 -> Add/1, Hydraulic Turbine and Governor/3
  wref/1 -> Hydraulic Turbine and Governor/1
  Vref/1 -> Excitation System/1
  Pref/1 -> Hydraulic Turbine and Governor/2
  Pe/1 -> Stabilizer/2(Pe), Hydraulic Turbine and Governor/4
  Excitation System/1 -> Vf/1
  Hydraulic Turbine and Governor/1 -> Stabilizer/1(Pm), Pm/1
  Hydraulic Turbine and Governor/2 -> Terminator/1

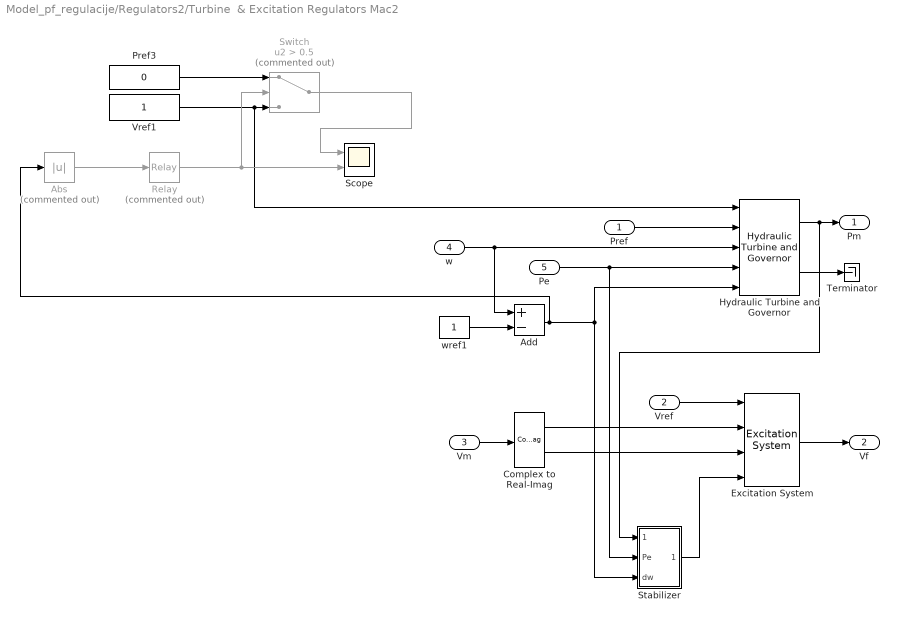
== system Model_pf_regulacije/Regulators2/Turbine  & Excitation Regulators Mac2 ==
  Pref : Inport
  Vref : Inport  Port=2
  Vm : Inport  Port=3
  w : Inport  Port=4
  Pe : Inport  Port=5
  Abs : Abs  Commented=on  SaturateOnIntegerOverflow=off
  Add : Sum  Inputs=+-
  Complex to Real-Imag : ComplexToRealImag
  Excitation System : spsExcitationSystemLib/Excitation System  tr=20e-3  reg=[ 300, 0.001 ]  exc=[ 1, 0 ]  tgr=[ 0, 0 ]  damp=[ 0.001, 0.1 ]  sat=[ 0, 0 ]  lim=[ -11.5, 11.5, 0 ]  v0=[1 1.3778]
  Hydraulic Turbine and Governor : spsHydraulicTurbineandGovernorLib/Hydraulic Turbine and Governor  sm="[ 10/3  0.07 ]"  gate="[  0.01  0.97518  -0.1  0.1 ]"  reg="[  0.05 1.163  0.105  0  0.01  ]"  hyd="[  0  2.67  ]"  dref=0  po=0.8201
  Pref3 : Constant  Value=0
  Relay : Relay  Commented=on  OnSwitchValue=0.04  OffSwitchValue=-1  OnOutputValue=0.5
  Scope : Scope  NumInputPorts=2
  Stabilizer : Subsystem
  Switch : Switch  Commented=on  Criteria=u2 > Threshold  Threshold=0.5  SaturateOnIntegerOverflow=off  InputSameDT=off
  Terminator : Terminator
  Vref1 : Constant
  wref1 : Constant
  Pm : Outport  VectorParamsAs1DForOutWhenUnconnected=off
  Vf : Outport  Port=2  VectorParamsAs1DForOutWhenUnconnected=off
  wires:
  Hydraulic Turbine and Governor/2 -> Terminator/1
  Hydraulic Turbine and Governor/1 -> Pm/1, Stabilizer/1(Pm)
  Excitation System/1 -> Vf/1
  Pe/1 -> Hydraulic Turbine and Governor/4, Stabilizer/2(Pe)
  Pref/1 -> Hydraulic Turbine and Governor/2
  Vref/1 -> Excitation System/1
  Switch/1 -> Scope/1
  w/1 -> Hydraulic Turbine and Governor/3, Add/1
  Vm/1 -> Complex to Real-Imag/1
  Complex to Real-Imag/2 -> Excitation System/3
  Complex to Real-Imag/1 -> Excitation System/2
  wref1/1 -> Add/2
  Add/1 -> Abs/1, Hydraulic Turbine and Governor/5, Stabilizer/3(dw)
  Stabilizer/1(Stab) -> Excitation System/4
  Vref1/1 -> Hydraulic Turbine and Governor/1, Switch/3
  Relay/1 -> Scope/2, Switch/2
  Abs/1 -> Relay/1
  Pref3/1 -> Switch/1

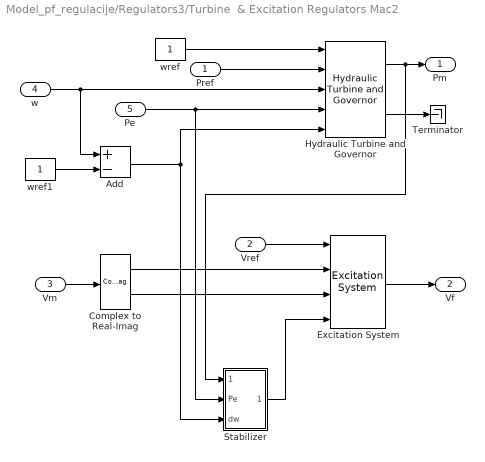
== system Model_pf_regulacije/Regulators3/Turbine  & Excitation Regulators Mac2 ==
  Pref : Inport
  Vref : Inport  Port=2
  Vm : Inport  Port=3
  w : Inport  Port=4
  Pe : Inport  Port=5
  Add : Sum  Inputs=+-
  Complex to Real-Imag : ComplexToRealImag
  Excitation System : spsExcitationSystemLib/Excitation System  tr=20e-3  reg=[ 300, 0.001 ]  exc=[ 1, 0 ]  tgr=[ 0, 0 ]  damp=[ 0.001, 0.1 ]  sat=[ 0, 0 ]  lim=[ -11.5, 11.5, 0 ]  v0=[1 1.4045]
  Hydraulic Turbine and Governor : spsHydraulicTurbineandGovernorLib/Hydraulic Turbine and Governor  sm="[ 10/3  0.07 ]"  gate="[  0.01  0.97518  -0.1  0.1 ]"  reg="[  0.05 1.163  0.105  0  0.01  ]"  hyd="[  0  2.67  ]"  dref=0  po=0.90231
  Stabilizer : Subsystem
  Terminator : Terminator
  wref : Constant
  wref1 : Constant
  Pm : Outport  VectorParamsAs1DForOutWhenUnconnected=off
  Vf : Outport  Port=2  VectorParamsAs1DForOutWhenUnconnected=off
  wires:
  Stabilizer/1(Stab) -> Excitation System/4
  Add/1 -> Stabilizer/3(dw), Hydraulic Turbine and Governor/5
  wref1/1 -> Add/2
  Complex to Real-Imag/1 -> Excitation System/2
  Complex to Real-Imag/2 -> Excitation System/3
  Vm/1 -> Complex to Real-Imag/1
  w/1 -> Add/1, Hydraulic Turbine and Governor/3
  wref/1 -> Hydraulic Turbine and Governor/1
  Vref/1 -> Excitation System/1
  Pref/1 -> Hydraulic Turbine and Governor/2
  Pe/1 -> Stabilizer/2(Pe), Hydraulic Turbine and Governor/4
  Excitation System/1 -> Vf/1
  Hydraulic Turbine and Governor/1 -> Stabilizer/1(Pm), Pm/1
  Hydraulic Turbine and Governor/2 -> Terminator/1

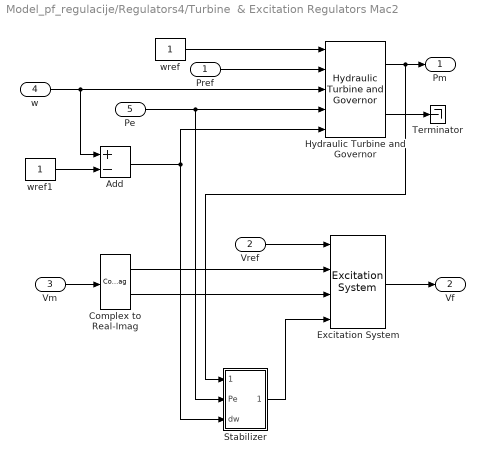
== system Model_pf_regulacije/Regulators4/Turbine  & Excitation Regulators Mac2 ==
  Pref : Inport
  Vref : Inport  Port=2
  Vm : Inport  Port=3
  w : Inport  Port=4
  Pe : Inport  Port=5
  Add : Sum  Inputs=+-
  Complex to Real-Imag : ComplexToRealImag
  Excitation System : spsExcitationSystemLib/Excitation System  tr=20e-3  reg=[ 300, 0.001 ]  exc=[ 1, 0 ]  tgr=[ 0, 0 ]  damp=[ 0.001, 0.1 ]  sat=[ 0, 0 ]  lim=[ -11.5, 11.5, 0 ]  v0=[1 1.4708]
  Hydraulic Turbine and Governor : spsHydraulicTurbineandGovernorLib/Hydraulic Turbine and Governor  sm="[ 10/3  0.07 ]"  gate="[  0.01  0.97518  -0.1  0.1 ]"  reg="[  0.05 1.163  0.105  0  0.01  ]"  hyd="[  0  2.67  ]"  dref=0  po=0.92838
  Stabilizer : Subsystem
  Terminator : Terminator
  wref : Constant
  wref1 : Constant
  Pm : Outport  VectorParamsAs1DForOutWhenUnconnected=off
  Vf : Outport  Port=2  VectorParamsAs1DForOutWhenUnconnected=off
  wires:
  Hydraulic Turbine and Governor/2 -> Terminator/1
  Hydraulic Turbine and Governor/1 -> Pm/1, Stabilizer/1(Pm)
  Excitation System/1 -> Vf/1
  Pe/1 -> Hydraulic Turbine and Governor/4, Stabilizer/2(Pe)
  Pref/1 -> Hydraulic Turbine and Governor/2
  Vref/1 -> Excitation System/1
  wref/1 -> Hydraulic Turbine and Governor/1
  w/1 -> Hydraulic Turbine and Governor/3, Add/1
  Vm/1 -> Complex to Real-Imag/1
  Complex to Real-Imag/2 -> Excitation System/3
  Complex to Real-Imag/1 -> Excitation System/2
  wref1/1 -> Add/2
  Add/1 -> Hydraulic Turbine and Governor/5, Stabilizer/3(dw)
  Stabilizer/1(Stab) -> Excitation System/4

== system Model_pf_regulacije/Regulators1/Turbine  & Excitation Regulators Mac2/Stabilizer ==
  Pm : Inport
  Pe : Inport  Port=2
  dw : Inport  Port=3
  Generic Power System Stabilizer : spsGenericPowerSystemStabilizerLib/Generic Power System Stabilizer  Tsensor=15e-3  K=2.5  Twashout=1  Tleadlag1="[0.06  1]"  Tleadlag2="[0  0]"  VSlimits=[-0.15 0.15]  Vinit=0  Plot_On=off  MagdB_On=on  FreqRange=logspace(-2,2,500)
  Ground1 : Ground
  Multi-Band Power System Stabilizer : spsMultiBandPowerSystemStabilizerLib/Multi-Band Power System Stabilizer  OperationMode=Simplified settings  Kg=0.7  GL=[0.2 10]  GI=[0.9 30]  GH=[12.0 115]  GLd=[66 66 9.4]  TcLF=[1.667 2 0 0 0 0 2 2.4 0 0 0 0 1 1]  GId=[66 66 47.6]  TcIF=[1 1 0.25 0.3 0 0 1 1 0.3 0.36 0 0 0 0]  GHd=[66 66 233]  TcHF="[0.01 0.012 0 0 0 0  0.012 0.0144 0 0 0 0 1 1]"  LIM=[.075 .15 .15 .15]  Plot_On=off  MagdB_On=on  FreqRange=logspace(-2,2,500)
  Multiport Switch : MultiPortSwitch
  PSS1 : Constant  Value=PSStype
  Sum2 : Sum  Inputs=+-  InputSameDT=on  SaturateOnIntegerOverflow=on  OutDataTypeStr=Inherit: Same as first input
  Stab : Outport  InitialOutput=0  VectorParamsAs1DForOutWhenUnconnected=off
  wires:
  PSS1/1 -> Multiport Switch/1
  Multi-Band Power System Stabilizer/1 -> Multiport Switch/4
  dw/1 -> Multi-Band Power System Stabilizer/1
  Ground1/1 -> Multiport Switch/2
  Pe/1 -> Sum2/2
  Pm/1 -> Sum2/1
  Sum2/1 -> Generic Power System Stabilizer/1
  Generic Power System Stabilizer/1 -> Multiport Switch/3
  Multiport Switch/1 -> Stab/1

== system Model_pf_regulacije/Regulators2/Turbine  & Excitation Regulators Mac2/Stabilizer ==
  Pm : Inport
  Pe : Inport  Port=2
  dw : Inport  Port=3
  Generic Power System Stabilizer : spsGenericPowerSystemStabilizerLib/Generic Power System Stabilizer  Tsensor=15e-3  K=2.5  Twashout=1  Tleadlag1="[0.06  1]"  Tleadlag2="[0  0]"  VSlimits=[-0.15 0.15]  Vinit=0  Plot_On=off  MagdB_On=on  FreqRange=logspace(-2,2,500)
  Ground1 : Ground
  Multi-Band Power System Stabilizer : spsMultiBandPowerSystemStabilizerLib/Multi-Band Power System Stabilizer  OperationMode=Simplified settings  Kg=0.7  GL=[0.2 10]  GI=[0.9 30]  GH=[12.0 115]  GLd=[66 66 9.4]  TcLF=[1.667 2 0 0 0 0 2 2.4 0 0 0 0 1 1]  GId=[66 66 47.6]  TcIF=[1 1 0.25 0.3 0 0 1 1 0.3 0.36 0 0 0 0]  GHd=[66 66 233]  TcHF="[0.01 0.012 0 0 0 0  0.012 0.0144 0 0 0 0 1 1]"  LIM=[.075 .15 .15 .15]  Plot_On=off  MagdB_On=on  FreqRange=logspace(-2,2,500)
  Multiport Switch : MultiPortSwitch
  PSS1 : Constant  Value=PSStype
  Sum2 : Sum  Inputs=+-  InputSameDT=on  SaturateOnIntegerOverflow=on  OutDataTypeStr=Inherit: Same as first input
  Stab : Outport  InitialOutput=0  VectorParamsAs1DForOutWhenUnconnected=off
  wires:
  Multi-Band Power System Stabilizer/1 -> Multiport Switch/4
  Multiport Switch/1 -> Stab/1
  Generic Power System Stabilizer/1 -> Multiport Switch/3
  Sum2/1 -> Generic Power System Stabilizer/1
  Pm/1 -> Sum2/1
  Pe/1 -> Sum2/2
  Ground1/1 -> Multiport Switch/2
  PSS1/1 -> Multiport Switch/1
  dw/1 -> Multi-Band Power System Stabilizer/1
